simulink model "prob"  (R2018b)
settings: Solver=VariableStepAuto  StartTime=0.0  StopTime=10  RelTol=1e-3
values from neighbouring files (symbols this model uses):
  delta_ksi = (20-(-20))/(2*r-1)    (= 1.37931034483)    [Parameter_S205.m]
  h = 0.4*10^(-3)    (= 0.0004)    [Parameter_S205.m]
  ksi = linspace(-20,20,2*r)    [Parameter_S205.m]
  l1 = 3.3    [Parameter_S205.m]
  l2 = 2.6    [Parameter_S205.m]
  l4 = 98    [Parameter_S205.m]
  sigma_norm = 1.6    [Parameter_S205.m]
settings Model: Creator=LENOVO  LastModifiedBy=LENOVO

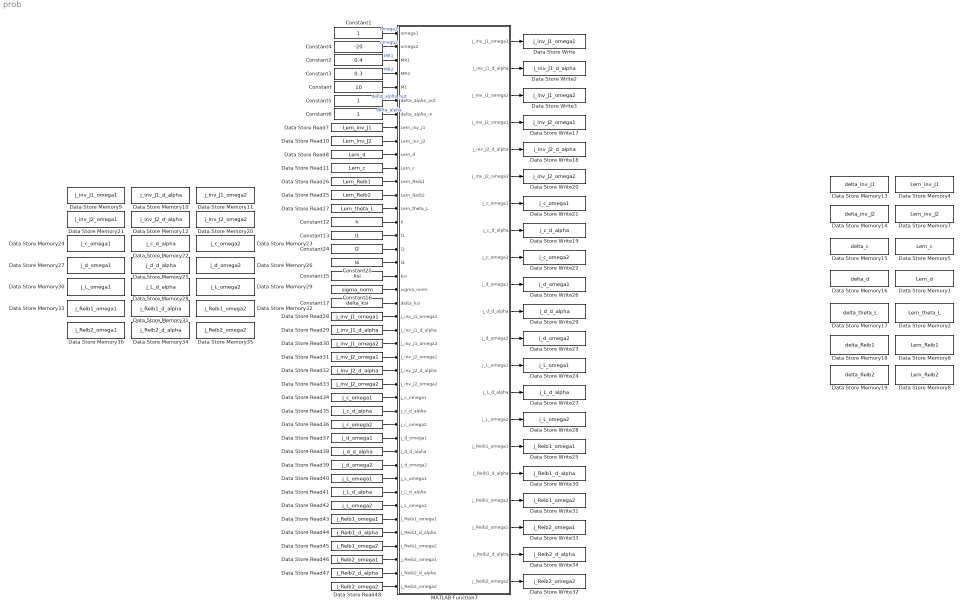
== system prob ==
  Constant : Constant  Value=10
  Constant1 : Constant
  Constant12 : Constant  Value=h
  Constant13 : Constant  Value=l1
  Constant15 : Constant  Value=ksi
  Constant16 : Constant  Value=sigma_norm
  Constant17 : Constant  Value=delta_ksi
  Constant2 : Constant  Value=0.4
  Constant24 : Constant  Value=l2
  Constant25 : Constant  Value=l4
  Constant3 : Constant  Value=0.3
  Constant4 : Constant  Value=-20
  Constant5 : Constant
  Constant6 : Constant
  Data Store Memory1 : DataStoreMemory  DataStoreName=Lern_d  ReadBeforeWriteMsg=warning  WriteAfterWriteMsg=warning  WriteAfterReadMsg=warning  InitialValue=1  ShowAdditionalParam=off
  Data Store Memory10 : DataStoreMemory  DataStoreName=j_inv_J1_d_alpha  ReadBeforeWriteMsg=warning  WriteAfterWriteMsg=warning  WriteAfterReadMsg=warning  ShowAdditionalParam=off
  Data Store Memory11 : DataStoreMemory  DataStoreName=j_inv_J1_omega2  ReadBeforeWriteMsg=warning  WriteAfterWriteMsg=warning  WriteAfterReadMsg=warning  ShowAdditionalParam=off
  Data Store Memory12 : DataStoreMemory  DataStoreName=j_inv_J2_d_alpha  ReadBeforeWriteMsg=warning  WriteAfterWriteMsg=warning  WriteAfterReadMsg=warning  ShowAdditionalParam=off
  Data Store Memory13 : DataStoreMemory  DataStoreName=delta_inv_J1  ReadBeforeWriteMsg=warning  WriteAfterWriteMsg=warning  WriteAfterReadMsg=warning  ShowAdditionalParam=off
  Data Store Memory14 : DataStoreMemory  DataStoreName=delta_inv_J2  ReadBeforeWriteMsg=warning  WriteAfterWriteMsg=warning  WriteAfterReadMsg=warning  ShowAdditionalParam=off
  Data Store Memory15 : DataStoreMemory  DataStoreName=delta_c  ReadBeforeWriteMsg=warning  WriteAfterWriteMsg=warning  WriteAfterReadMsg=warning  ShowAdditionalParam=off
  Data Store Memory16 : DataStoreMemory  DataStoreName=delta_d  ReadBeforeWriteMsg=warning  WriteAfterWriteMsg=warning  WriteAfterReadMsg=warning  ShowAdditionalParam=off
  Data Store Memory17 : DataStoreMemory  DataStoreName=delta_theta_L  ReadBeforeWriteMsg=warning  WriteAfterWriteMsg=warning  WriteAfterReadMsg=warning  ShowAdditionalParam=off
  Data Store Memory18 : DataStoreMemory  DataStoreName=delta_Reib1  ReadBeforeWriteMsg=warning  WriteAfterWriteMsg=warning  WriteAfterReadMsg=warning  InitialValue=zeros(1,30)  ShowAdditionalParam=off
  Data Store Memory19 : DataStoreMemory  DataStoreName=delta_Reib2  ReadBeforeWriteMsg=warning  WriteAfterWriteMsg=warning  WriteAfterReadMsg=warning  InitialValue=zeros(1,30)  ShowAdditionalParam=off
  Data Store Memory2 : DataStoreMemory  DataStoreName=Lern_theta_L  ReadBeforeWriteMsg=warning  WriteAfterWriteMsg=warning  WriteAfterReadMsg=warning  ShowAdditionalParam=off
  Data Store Memory20 : DataStoreMemory  DataStoreName=j_inv_J2_omega2  ReadBeforeWriteMsg=warning  WriteAfterWriteMsg=warning  WriteAfterReadMsg=warning  ShowAdditionalParam=off
  Data Store Memory21 : DataStoreMemory  DataStoreName=j_inv_J2_omega1  ReadBeforeWriteMsg=warning  WriteAfterWriteMsg=warning  WriteAfterReadMsg=warning  ShowAdditionalParam=off
  Data Store Memory22 : DataStoreMemory  DataStoreName=j_c_d_alpha  ReadBeforeWriteMsg=warning  WriteAfterWriteMsg=warning  WriteAfterReadMsg=warning  ShowAdditionalParam=off
  Data Store Memory23 : DataStoreMemory  DataStoreName=j_c_omega2  ReadBeforeWriteMsg=warning  WriteAfterWriteMsg=warning  WriteAfterReadMsg=warning  ShowAdditionalParam=off
  Data Store Memory24 : DataStoreMemory  DataStoreName=j_c_omega1  ReadBeforeWriteMsg=warning  WriteAfterWriteMsg=warning  WriteAfterReadMsg=warning  ShowAdditionalParam=off
  Data Store Memory25 : DataStoreMemory  DataStoreName=j_d_d_alpha  ReadBeforeWriteMsg=warning  WriteAfterWriteMsg=warning  WriteAfterReadMsg=warning  ShowAdditionalParam=off
  Data Store Memory26 : DataStoreMemory  DataStoreName=j_d_omega2  ReadBeforeWriteMsg=warning  WriteAfterWriteMsg=warning  WriteAfterReadMsg=warning  ShowAdditionalParam=off
  Data Store Memory27 : DataStoreMemory  DataStoreName=j_d_omega1  ReadBeforeWriteMsg=warning  WriteAfterWriteMsg=warning  WriteAfterReadMsg=warning  ShowAdditionalParam=off
  Data Store Memory28 : DataStoreMemory  DataStoreName=j_L_d_alpha  ReadBeforeWriteMsg=warning  WriteAfterWriteMsg=warning  WriteAfterReadMsg=warning  ShowAdditionalParam=off
  Data Store Memory29 : DataStoreMemory  DataStoreName=j_L_omega2  ReadBeforeWriteMsg=warning  WriteAfterWriteMsg=warning  WriteAfterReadMsg=warning  ShowAdditionalParam=off
  Data Store Memory30 : DataStoreMemory  DataStoreName=j_L_omega1  ReadBeforeWriteMsg=warning  WriteAfterWriteMsg=warning  WriteAfterReadMsg=warning  ShowAdditionalParam=off
  Data Store Memory31 : DataStoreMemory  DataStoreName=j_Reib1_d_alpha  ReadBeforeWriteMsg=warning  WriteAfterWriteMsg=warning  WriteAfterReadMsg=warning  InitialValue=zeros(1,30)  ShowAdditionalParam=off
  Data Store Memory32 : DataStoreMemory  DataStoreName=j_Reib1_omega2  ReadBeforeWriteMsg=warning  WriteAfterWriteMsg=warning  WriteAfterReadMsg=warning  InitialValue=zeros(1,30)  ShowAdditionalParam=off
  Data Store Memory33 : DataStoreMemory  DataStoreName=j_Reib1_omega1  ReadBeforeWriteMsg=warning  WriteAfterWriteMsg=warning  WriteAfterReadMsg=warning  InitialValue=zeros(1,30)  ShowAdditionalParam=off
  Data Store Memory34 : DataStoreMemory  DataStoreName=j_Reib2_d_alpha  ReadBeforeWriteMsg=warning  WriteAfterWriteMsg=warning  WriteAfterReadMsg=warning  InitialValue=zeros(1,30)  ShowAdditionalParam=off
  Data Store Memory35 : DataStoreMemory  DataStoreName=j_Reib2_omega2  ReadBeforeWriteMsg=warning  WriteAfterWriteMsg=warning  WriteAfterReadMsg=warning  InitialValue=zeros(1,30)  ShowAdditionalParam=off
  Data Store Memory36 : DataStoreMemory  DataStoreName=j_Reib2_omega1  ReadBeforeWriteMsg=warning  WriteAfterWriteMsg=warning  WriteAfterReadMsg=warning  InitialValue=zeros(1,30)  ShowAdditionalParam=off
  Data Store Memory4 : DataStoreMemory  DataStoreName=Lern_inv_J1  ReadBeforeWriteMsg=warning  WriteAfterWriteMsg=warning  WriteAfterReadMsg=warning  InitialValue=0.2  ShowAdditionalParam=off
  Data Store Memory5 : DataStoreMemory  DataStoreName=Lern_c  ReadBeforeWriteMsg=warning  WriteAfterWriteMsg=warning  WriteAfterReadMsg=warning  InitialValue=1350  ShowAdditionalParam=off
  Data Store Memory6 : DataStoreMemory  DataStoreName=Lern_Reib1  ReadBeforeWriteMsg=warning  WriteAfterWriteMsg=warning  WriteAfterReadMsg=warning  InitialValue=zeros(1,30)  ShowAdditionalParam=off
  Data Store Memory7 : DataStoreMemory  DataStoreName=Lern_inv_J2  ReadBeforeWriteMsg=warning  WriteAfterWriteMsg=warning  WriteAfterReadMsg=warning  InitialValue=0.45  ShowAdditionalParam=off
  Data Store Memory8 : DataStoreMemory  DataStoreName=Lern_Reib2  ReadBeforeWriteMsg=warning  WriteAfterWriteMsg=warning  WriteAfterReadMsg=warning  InitialValue=zeros(1,30)  ShowAdditionalParam=off
  Data Store Memory9 : DataStoreMemory  DataStoreName=j_inv_J1_omega1  ReadBeforeWriteMsg=warning  WriteAfterWriteMsg=warning  WriteAfterReadMsg=warning  ShowAdditionalParam=off
  Data Store Read10 : DataStoreRead  DataStoreName=Lern_inv_J2
  Data Store Read11 : DataStoreRead  DataStoreName=Lern_c
  Data Store Read25 : DataStoreRead  DataStoreName=Lern_Reib2
  Data Store Read26 : DataStoreRead  DataStoreName=Lern_Reib1
  Data Store Read27 : DataStoreRead  DataStoreName=Lern_theta_L
  Data Store Read28 : DataStoreRead  DataStoreName=j_inv_J1_omega1
  Data Store Read29 : DataStoreRead  DataStoreName=j_inv_J1_d_alpha
  Data Store Read30 : DataStoreRead  DataStoreName=j_inv_J1_omega2
  Data Store Read31 : DataStoreRead  DataStoreName=j_inv_J2_omega1
  Data Store Read32 : DataStoreRead  DataStoreName=j_inv_J2_d_alpha
  Data Store Read33 : DataStoreRead  DataStoreName=j_inv_J2_omega2
  Data Store Read34 : DataStoreRead  DataStoreName=j_c_omega1
  Data Store Read35 : DataStoreRead  DataStoreName=j_c_d_alpha
  Data Store Read36 : DataStoreRead  DataStoreName=j_c_omega2
  Data Store Read37 : DataStoreRead  DataStoreName=j_d_omega1
  Data Store Read38 : DataStoreRead  DataStoreName=j_d_d_alpha
  Data Store Read39 : DataStoreRead  DataStoreName=j_d_omega2
  Data Store Read40 : DataStoreRead  DataStoreName=j_L_omega1
  Data Store Read41 : DataStoreRead  DataStoreName=j_L_d_alpha
  Data Store Read42 : DataStoreRead  DataStoreName=j_L_omega2
  Data Store Read43 : DataStoreRead  DataStoreName=j_Reib1_omega1
  Data Store Read44 : DataStoreRead  DataStoreName=j_Reib1_d_alpha
  Data Store Read45 : DataStoreRead  DataStoreName=j_Reib1_omega2
  Data Store Read46 : DataStoreRead  DataStoreName=j_Reib2_omega1
  Data Store Read47 : DataStoreRead  DataStoreName=j_Reib2_d_alpha
  Data Store Read48 : DataStoreRead  DataStoreName=j_Reib2_omega2
  Data Store Read7 : DataStoreRead  DataStoreName=Lern_inv_J1
  Data Store Read8 : DataStoreRead  DataStoreName=Lern_d
  Data Store Write : DataStoreWrite  DataStoreName=j_inv_J1_omega1
  Data Store Write17 : DataStoreWrite  DataStoreName=j_inv_J2_omega1
  Data Store Write18 : DataStoreWrite  DataStoreName=j_inv_J2_d_alpha
  Data Store Write19 : DataStoreWrite  DataStoreName=j_c_d_alpha
  Data Store Write2 : DataStoreWrite  DataStoreName=j_inv_J1_d_alpha
  Data Store Write20 : DataStoreWrite  DataStoreName=j_inv_J2_omega2
  Data Store Write21 : DataStoreWrite  DataStoreName=j_c_omega1
  Data Store Write22 : DataStoreWrite  DataStoreName=j_c_omega2
  Data Store Write23 : DataStoreWrite  DataStoreName=j_d_omega2
  Data Store Write24 : DataStoreWrite  DataStoreName=j_L_omega1
  Data Store Write25 : DataStoreWrite  DataStoreName=j_Reib1_omega1
  Data Store Write26 : DataStoreWrite  DataStoreName=j_d_omega1
  Data Store Write27 : DataStoreWrite  DataStoreName=j_L_d_alpha
  Data Store Write28 : DataStoreWrite  DataStoreName=j_L_omega2
  Data Store Write29 : DataStoreWrite  DataStoreName=j_d_d_alpha
  Data Store Write3 : DataStoreWrite  DataStoreName=j_inv_J1_omega2
  Data Store Write30 : DataStoreWrite  DataStoreName=j_Reib1_d_alpha
  Data Store Write31 : DataStoreWrite  DataStoreName=j_Reib1_omega2
  Data Store Write32 : DataStoreWrite  DataStoreName=j_Reib2_omega2
  Data Store Write33 : DataStoreWrite  DataStoreName=j_Reib2_omega1
  Data Store Write34 : DataStoreWrite  DataStoreName=j_Reib2_d_alpha
  MATLAB Function7 : MATLAB Function  TreatAsAtomicUnit=on
  wires:
  Data Store Read27/1 -> MATLAB Function7/14(Lern_theta_L)
  Data Store Read37/1 -> MATLAB Function7/31("j_d_omega1 ")
  Data Store Read40/1 -> MATLAB Function7/34("j_L_omega1 ")
  Data Store Read29/1 -> MATLAB Function7/23("j_inv_J1_d_alpha ")
  Data Store Read25/1 -> MATLAB Function7/13(Lern_Reib2)
  MATLAB Function7/11(j_d_d_alpha) -> Data Store Write29/1
  Constant25/1 -> MATLAB Function7/18(l4)
  Data Store Read11/1 -> MATLAB Function7/11(Lern_c)
  MATLAB Function7/10(j_d_omega1) -> Data Store Write26/1
  MATLAB Function7/5(j_inv_J2_d_alpha) -> Data Store Write18/1
  MATLAB Function7/7(j_c_omega1) -> Data Store Write21/1
  MATLAB Function7/9(j_c_omega2) -> Data Store Write22/1
  MATLAB Function7/17(j_Reib1_d_alpha) -> Data Store Write30/1
  Constant17/1 -> MATLAB Function7/21(delta_ksi)
  MATLAB Function7/16(j_Reib1_omega1) -> Data Store Write25/1
  Data Store Read41/1 -> MATLAB Function7/35("j_L_d_alpha ")
  Data Store Read26/1 -> MATLAB Function7/12(Lern_Reib1)
  MATLAB Function7/15(j_L_omega2) -> Data Store Write28/1
  MATLAB Function7/18(j_Reib1_omega2) -> Data Store Write31/1
  Data Store Read32/1 -> MATLAB Function7/26("j_inv_J2_d_alpha ")
  MATLAB Function7/20(j_Reib2_d_alpha) -> Data Store Write34/1
  Data Store Read34/1 -> MATLAB Function7/28("j_c_omega1 ")
  MATLAB Function7/21(j_Reib2_omega2) -> Data Store Write32/1
  Data Store Read47/1 -> MATLAB Function7/41("j_Reib2_d_alpha ")
  Data Store Read48/1 -> MATLAB Function7/42("j_Reib2_omega2 ")
  MATLAB Function7/13(j_L_omega1) -> Data Store Write24/1
  Data Store Read44/1 -> MATLAB Function7/38("j_Reib1_d_alpha ")
  Constant24/1 -> MATLAB Function7/17(l2)
  MATLAB Function7/6(j_inv_J2_omega2) -> Data Store Write20/1
  Data Store Read36/1 -> MATLAB Function7/30("j_c_omega2 ")
  Data Store Read10/1 -> MATLAB Function7/9(Lern_inv_J2)
  Data Store Read46/1 -> MATLAB Function7/40("j_Reib2_omega1 ")
  Constant6/1 -> MATLAB Function7/7(delta_alpha_in)  "delta_alpha"
  Data Store Read7/1 -> MATLAB Function7/8(Lern_inv_J1)
  Data Store Read43/1 -> MATLAB Function7/37("j_Reib1_omega1 ")
  Data Store Read38/1 -> MATLAB Function7/32("j_d_d_alpha ")
  Data Store Read33/1 -> MATLAB Function7/27("j_inv_J2_omega2 ")
  MATLAB Function7/19(j_Reib2_omega1) -> Data Store Write33/1
  Constant15/1 -> MATLAB Function7/19(ksi)
  Data Store Read8/1 -> MATLAB Function7/10(Lern_d)
  Data Store Read45/1 -> MATLAB Function7/39("j_Reib1_omega2 ")
  Data Store Read35/1 -> MATLAB Function7/29("j_c_d_alpha ")
  Constant2/1 -> MATLAB Function7/3(MR1)  "MR1"
  Data Store Read31/1 -> MATLAB Function7/25("j_inv_J2_omega1 ")
  MATLAB Function7/12(j_d_omega2) -> Data Store Write23/1
  Constant13/1 -> MATLAB Function7/16(l1)
  MATLAB Function7/14(j_L_d_alpha) -> Data Store Write27/1
  MATLAB Function7/3(j_inv_J1_omega2) -> Data Store Write3/1
  Constant12/1 -> MATLAB Function7/15(h)
  Data Store Read28/1 -> MATLAB Function7/22("j_inv_J1_omega1 ")
  Constant1/1 -> MATLAB Function7/1(omega1)  "omega1"
  Constant16/1 -> MATLAB Function7/20(sigma_norm)
  MATLAB Function7/2(j_inv_J1_d_alpha) -> Data Store Write2/1
  MATLAB Function7/8(j_c_d_alpha) -> Data Store Write19/1
  Data Store Read39/1 -> MATLAB Function7/33("j_d_omega2 ")
  MATLAB Function7/4(j_inv_J2_omega1) -> Data Store Write17/1
  Data Store Read42/1 -> MATLAB Function7/36("j_L_omega2 ")
  Constant4/1 -> MATLAB Function7/2(omega2)  "omega2"
  MATLAB Function7/1(j_inv_J1_omega1) -> Data Store Write/1
  Constant5/1 -> MATLAB Function7/6(delta_alpha_out)  "delta_alpha_out"
  Data Store Read30/1 -> MATLAB Function7/24("j_inv_J1_omega2 ")
  Constant3/1 -> MATLAB Function7/4(MR2)  "MR2"
  Constant/1 -> MATLAB Function7/5(M1)

== matlab function prob/MATLAB Function7 ==
  data: omega1 input; omega2 input; MR1 input; MR2 input; M1 input; delta_alpha_out input; delta_alpha_in input; j_inv_J1_omega1 output; Lern_inv_J1 input; Lern_inv_J2 input; Lern_d input; Lern_c input; Lern_Reib1 input; Lern_Reib2 input; Lern_theta_L input; j_inv_J1_d_alpha output; h input; l1 input; l2 input; l4 input; ksi input; sigma_norm input; delta_ksi input; j_inv_J1_omega2 output; j_inv_J2_omega1 output; j_inv_J2_d_alpha output; j_inv_J2_omega2 output; j_c_omega1 output; j_c_d_alpha output; j_c_omega2 output; j_d_omega1 output; j_d_d_alpha output; j_d_omega2 output; j_L_omega1 output; j_L_d_alpha output; j_L_omega2 output; j_Reib1_omega1 output; j_Reib1_d_alpha output; j_Reib1_omega2 output; j_Reib2_omega1 output; j_Reib2_d_alpha output; j_Reib2_omega2 output; j_inv_J1_omega1 input; j_inv_J1_d_alpha input; j_inv_J1_omega2 input; j_inv_J2_omega1 input; j_inv_J2_d_alpha input; j_inv_J2_omega2 input; j_c_omega1 input; j_c_d_alpha input; j_c_omega2 input; j_d_omega1 input; j_d_d_alpha input; j_d_omega2 input; j_L_omega1 input; j_L_d_alpha input; j_L_omega2 input; j_Reib1_omega1 input; j_Reib1_d_alpha input; j_Reib1_omega2 input; j_Reib2_omega1 input; j_Reib2_d_alpha input; j_Reib2_omega2 input
function [j_inv_J1_omega1,j_inv_J1_d_alpha,j_inv_J1_omega2,j_inv_J2_omega1,j_inv_J2_d_alpha,j_inv_J2_omega2,j_c_omega1,j_c_d_alpha,j_c_omega2,j_d_omega1,j_d_d_alpha,j_d_omega2,j_L_omega1,j_L_d_alpha,j_L_omega2,j_Reib1_omega1,j_Reib1_d_alpha,j_Reib1_omega2,j_Reib2_omega1,j_Reib2_d_alpha,j_Reib2_omega2]=Partielle_Ableitung(omega1,omega2,MR1,MR2,M1,delta_alpha_out,delta_alpha_in,Lern_inv_J1,Lern_inv_J2,Lern_d,Lern_c,Lern_Reib1,Lern_Reib2,Lern_theta_L,h,l1,l2,l4,ksi,sigma_norm,delta_ksi,j_inv_J1_omega1,j_inv_J1_d_alpha,j_inv_J1_omega2,j_inv_J2_omega1,j_inv_J2_d_alpha,j_inv_J2_omega2,j_c_omega1,j_c_d_alpha,j_c_omega2,j_d_omega1,j_d_d_alpha,j_d_omega2,j_L_omega1,j_L_d_alpha,j_L_omega2,j_Reib1_omega1,j_Reib1_d_alpha,j_Reib1_omega2,j_Reib2_omega1,j_Reib2_d_alpha,j_Reib2_omega2)

% Aktivierungsfunktionen
Zaehler_AF_GRNN=@(u,ksi) exp(-(u-ksi).^2/(2*sigma_norm^2*delta_ksi^2));
Nenner_AF_GRNN=@(u,ksi) sum(Zaehler_AF_GRNN(u,ksi));
AF_GRNN=@(u,ksi) Zaehler_AF_GRNN(u,ksi)/Nenner_AF_GRNN(u,ksi);

% partielle Ableitung des Reibapproximators
Grad_Reib1=0;
for j=1:30
    Grad_Reib1=Grad_Reib1+AF_GRNN(omega1,ksi(j))*(omega1-ksi(j))/(sigma_norm^2*delta_ksi^2)*(MR1-Lern_Reib1(j));
end

Grad_Reib2=0;
for j=1:30
    Grad_Reib2=Grad_Reib2+AF_GRNN(omega2,ksi(j))*(omega2-ksi(j))/(sigma_norm^2*delta_ksi^2)*(MR2-Lern_Reib2(j));
end

% partielle Ableitung des Loseapproximators
Grad_alpha_out_inv_J1=0;
Grad_alpha_out_inv_J2=0;
Grad_alpha_out_c=0;
Grad_alpha_out_d=0;
Grad_alpha_out_Reib1=zeros(1,30);
Grad_alpha_out_Reib2=zeros(1,30);
Grad_alpha_out_L=0;

if delta_alpha_in>Lern_theta_L
    Grad_alpha_out_inv_J1=j_inv_J1_d_alpha;
    Grad_alpha_out_inv_J2=j_inv_J2_d_alpha;
    Grad_alpha_out_c=j_c_d_alpha;
    Grad_alpha_out_d=j_d_d_alpha;
    Grad_alpha_out_Reib1=j_Reib1_d_alpha;
    Grad_alpha_out_Reib2=j_Reib2_d_alpha;
    Grad_alpha_out_L=j_L_d_alpha-1;
elseif delta_alpha_in<-Lern_theta_L
    Grad_alpha_out_inv_J1=j_inv_J1_d_alpha;
    Grad_alpha_out_inv_J2=j_inv_J2_d_alpha;
    Grad_alpha_out_c=j_c_d_alpha;
    Grad_alpha_out_d=j_d_d_alpha;
    Grad_alpha_out_Reib1=j_Reib1_d_alpha;
    Grad_alpha_out_Reib2=j_Reib2_d_alpha;
    Grad_alpha_out_L=j_L_d_alpha+1;
else
    Grad_alpha_out_inv_J1=0;
    Grad_alpha_out_inv_J2=0;
    Grad_alpha_out_c=0;
    Grad_alpha_out_d=0;
    Grad_alpha_out_Reib1=zeros(1,30);
    Grad_alpha_out_Reib2=zeros(1,30);
    Grad_alpha_out_L=0;
end

% j-Parameter abhaengig von d_alpha
j_inv_J1_d_alpha=j_inv_J1_d_alpha+h*(l2+1)*j_inv_J1_omega1-h*j_inv_J1_omega2;
j_inv_J2_d_alpha=j_inv_J2_d_alpha+h*(l2+1)*j_inv_J2_omega1-h*j_inv_J2_omega2;
j_c_d_alpha=j_c_d_alpha+h*(l2+1)*j_c_omega1-h*j_c_omega2;
j_d_d_alpha=j_d_d_alpha+h*(l2+1)*j_d_omega1-h*j_d_omega2;
j_Reib1_d_alpha=j_Reib1_d_alpha+h.*(l2+1).*j_Reib1_omega1-h.*j_Reib1_omega2;
j_Reib2_d_alpha=j_Reib2_d_alpha+h.*(l2+1).*j_Reib2_omega1-h.*j_Reib2_omega2;
j_L_d_alpha=j_L_d_alpha+h*(l2+1)*j_L_omega1-h*j_L_omega2;

% j-Parameter abhaengig von omega2
j_inv_J1_omega2=j_inv_J1_omega2+h*l4*j_inv_J1_omega1-h*Lern_inv_J2*j_inv_J1_omega2*Grad_Reib2+(h*Lern_c*Lern_inv_J2+Lern_d*Lern_inv_J2)*Grad_alpha_out_inv_J1;
j_inv_J2_omega2=j_inv_J2_omega2+h*l4*j_inv_J2_omega1-h*MR2-h*Lern_inv_J2*j_inv_J2_omega2*Grad_Reib2+(h*Lern_c+Lern_d)*delta_alpha_out+(h*Lern_c*Lern_inv_J2+Lern_d*Lern_inv_J2)*Grad_alpha_out_inv_J2;
j_c_omega2=j_c_omega2+h*l4*j_c_omega1-h*Lern_inv_J2*j_c_omega2*Grad_Reib2+h*Lern_inv_J2*delta_alpha_out+(h*Lern_c*Lern_inv_J2+Lern_d*Lern_inv_J2)*Grad_alpha_out_c;
j_d_omega2=j_d_omega2+h*l4*j_d_omega1-h*Lern_inv_J2*j_d_omega2*Grad_Reib2+Lern_inv_J2*delta_alpha_out+(h*Lern_c*Lern_inv_J2+Lern_d*Lern_inv_J2)*Grad_alpha_out_d;
j_Reib1_omega2=j_Reib1_omega2+h.*l4.*j_Reib1_omega1-h.*Lern_inv_J2.*Grad_Reib2.*j_Reib1_omega2+(h.*Lern_c.*Lern_inv_J2+Lern_d.*Lern_inv_J2).*Grad_alpha_out_Reib1;
j_Reib2_omega2=j_Reib2_omega2+h.*l4.*j_Reib2_omega1-h.*Lern_inv_J2.*(AF_GRNN(omega2,ksi)+j_Reib2_omega2.*Grad_Reib2)+(h.*Lern_c.*Lern_inv_J2+Lern_d.*Lern_inv_J2).*Grad_alpha_out_Reib2;
j_L_omega2=j_L_omega2+h*l4*j_L_omega1-h*Lern_inv_J2*j_L_omega2*Grad_Reib2+(h*Lern_c*Lern_inv_J2+Lern_d*Lern_inv_J2)*Grad_alpha_out_L;

% j-Parameter abhaengig von omega1
j_inv_J1_omega1=(1+h*l1)*j_inv_J1_omega1+h*M1-h*MR1-h*Lern_inv_J1*j_inv_J1_omega1*Grad_Reib1-(h*Lern_c+Lern_d)*delta_alpha_out-(h*Lern_inv_J1*Lern_c+Lern_inv_J1*Lern_d)*Grad_alpha_out_inv_J1;
j_inv_J2_omega1=(1+h*l1)*j_inv_J2_omega1-h*Lern_inv_J1*j_inv_J2_omega1*Grad_Reib1-(h*Lern_inv_J1*Lern_c+Lern_inv_J1*Lern_d)*Grad_alpha_out_inv_J2;
j_c_omega1=(1+h*l1)*j_c_omega1-h*Lern_inv_J1*j_c_omega1*Grad_Reib1-h*Lern_inv_J1*delta_alpha_out-(h*Lern_inv_J1*Lern_c+Lern_inv_J1*Lern_d)*Grad_alpha_out_c;
j_d_omega1=(1+h*l1)*j_d_omega1-h*Lern_inv_J1*j_d_omega1*Grad_Reib1-Lern_inv_J1*delta_alpha_out-(h*Lern_inv_J1*Lern_c+Lern_inv_J1*Lern_d)*Grad_alpha_out_d;
j_Reib1_omega1=(1+h.*l1).*j_Reib1_omega1-h.*Lern_inv_J1.*(AF_GRNN(omega1,ksi)+j_Reib1_omega1.*Grad_Reib1)-(h.*Lern_inv_J1.*Lern_c+Lern_inv_J1.*Lern_d).*Grad_alpha_out_Reib1;
j_Reib2_omega1=(1+h.*l1).*j_Reib2_omega1-h.*Lern_inv_J1.*j_Reib2_omega1.*Grad_Reib1-(h.*Lern_inv_J1.*Lern_c+Lern_inv_J1.*Lern_d).*Grad_alpha_out_Reib2;
j_L_omega1=(1+h*l1)*j_L_omega1-h*Lern_inv_J1*j_L_omega1*Grad_Reib1-(h*Lern_inv_J1*Lern_c+Lern_inv_J1*Lern_d)*Grad_alpha_out_L;

end
